simulink model "City_Env_2Car_TS2020"  (Simulink 8.5)
settings: Solver=ode45  StartTime=0.0  StopTime=120  RelTol=1e-3
libraries: Solver_SF x2
settings Model: Creator=elowe  LastModifiedBy=mkhan  CovHtmlReporting=off  CovSFcnEnable=off
settings DebuggingCC: SolverPrmCheckMsg=warning  FcnCallInpInsideContextMsg=EnableAllAsWarning
settings GRTTargetCC: CombineOutputUpdateFcns=on  GRTInterface=off

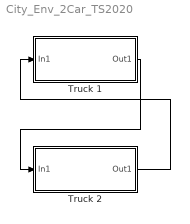
== system City_Env_2Car_TS2020 ==
  Truck 1 : Subsystem
  Truck 2 : Subsystem
  wires:
  Truck 1/1(Out1) -> Truck 2/1(In1)
  Truck 2/1(Out1) -> Truck 1/1(In1)

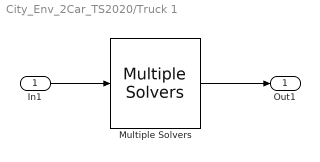
== system City_Env_2Car_TS2020/Truck 1 ==
  In1 : Inport
  Multiple Solvers : Solver_SF/Multiple Solvers  Priority=1  iVehicle=1  SIMFILE=D:\product_dev\trunk\Image\TruckSim\Core\TruckSim_Data\Extensions\Simulink\Multi_Vehicle\simfile1.sim  Run_RTs=off  vs_state_ind=Run  StopMode_ind=Vehicle Model  vs_scx=on
  Out1 : Outport
  wires:
  In1/1 -> Multiple Solvers/1
  Multiple Solvers/1 -> Out1/1

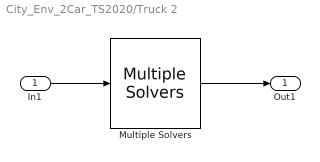
== system City_Env_2Car_TS2020/Truck 2 ==
  In1 : Inport
  Multiple Solvers : Solver_SF/Multiple Solvers  Priority=1  iVehicle=2  SIMFILE=D:\product_dev\trunk\Image\TruckSim\Core\TruckSim_Data\Extensions\Simulink\Multi_Vehicle\simfile2.sim  Run_RTs=off  vs_state_ind=Run  StopMode_ind=Vehicle Model  vs_scx=on
  Out1 : Outport
  wires:
  In1/1 -> Multiple Solvers/1
  Multiple Solvers/1 -> Out1/1
